simulink model "MMC_SwitchingModel_20250511"  (R2024b)
settings: Solver=VariableStepAuto  StartTime=0.0  StopTime=0.35  RelTol=1e-3
values from neighbouring files (symbols this model uses):
  Ceq = 3e-3    (= 0.003)    [param_allsim_20250429.m]
  f0 = 50    [param_allsim_20250429.m]
  Fc = 1e3    (= 1000)    [param_allsim_20250429.m]
  L_ac = 100e-6    (= 0.0001)    [param_allsim_20250429.m]
  L_arm = 1e-3    (= 0.001)    [param_allsim_20250429.m]
  m_Delta_0 = m_Delta_0_n    (= 0)    [param_allsim_20250429.m]
  m_Delta_d = M_Delta*sin(Phi_Delta)    [param_allsim_20250429.m]
  m_Delta_q = -M_Delta*cos(Phi_Delta)    [param_allsim_20250429.m]
  m_Sigma_0 = m_Sigma_0_n    (= 1)    [param_allsim_20250429.m]
  m_Sigma_d = M_Sigma*sin(Phi_Sigma)    [param_allsim_20250429.m]
  m_Sigma_q = -M_Sigma*cos(Phi_Sigma)    [param_allsim_20250429.m]
  N = 6    [param_allsim_20250429.m]
  R_ac = 1    [param_allsim_20250429.m]
  R_arm = 1e-2    (= 0.01)    [param_allsim_20250429.m]
  VDC = 800    [param_allsim_20250429.m]
undefined symbols (not defined in the file or in its folder): C_SM
libraries: spsVoltageMeasurementLib x11, spsCurrentMeasurementLib x8, spsSeriesRLCBranchLib x6, spsHalfBridgeMMCLib x6, spsPWMGeneratorMultilevelLib x6, spsabctodq0Lib x6, spsDCVoltageSourceLib x2, spsdq0toabcLib x2, spsGroundLib x1, spsThreePhaseSeriesRLCBranchLib x1, spsMeanLib x1, spspowerguiLib x1
(part 2 of 2)

== matlab function MMC_SwitchingModel_20250511/ /Sinus Modulation + Sorting Algorithm/Subsystem3/MATLAB Function1 ==
  data: ordre input; y output; sens input; N_on input
function y = fcn(ordre,sens,N_on)

N_m = length(ordre);
Gp = zeros(1,2*N_m);
Ap0=ordre;

%% Sens positif (sens = 1)
if sens==1         % ON les condensateurs les moins chargés
    
    %K1 = 1 ; K2 = 0
    kp = 1:N_on;
    Gp(2*Ap0(kp))=0;
    Gp(2*Ap0(kp)-1)=1;
    
    %K1 = 0 ; K2 = 1
    kp = N_on+1:N_m;
    Gp(2*Ap0(kp))=1;
    Gp(2*Ap0(kp)-1)=0;

else            % ON les condensateurs les plus chargés
    
    %K1 = 1 ; K2 = 0
    kp = N_m:-1:N_m+1-N_on;
    Gp(2*Ap0(kp))=0;
    Gp(2*Ap0(kp)-1)=1;
    
    %K1 = 0 ; K2 = 1
    kp = N_m-N_on:-1:1;
    Gp(2*Ap0(kp))=1;
    Gp(2*Ap0(kp)-1)=0;
end
y=Gp;

== matlab function MMC_SwitchingModel_20250511/ /Sinus Modulation + Sorting Algorithm/Subsystem3/MATLAB Function2 ==
  data: ordre input; y output; sens input; N_on input
function y = fcn(ordre,sens,N_on)

N_m = length(ordre);
Gp = zeros(1,2*N_m);
Ap0=ordre;

%% Sens positif (sens = 1)
if sens==1         % ON les condensateurs les moins chargés
    
    %K1 = 1 ; K2 = 0
    kp = 1:N_on;
    Gp(2*Ap0(kp))=0;
    Gp(2*Ap0(kp)-1)=1;
    
    %K1 = 0 ; K2 = 1
    kp = N_on+1:N_m;
    Gp(2*Ap0(kp))=1;
    Gp(2*Ap0(kp)-1)=0;

else            % ON les condensateurs les plus chargés
    
    %K1 = 1 ; K2 = 0
    kp = N_m:-1:N_m+1-N_on;
    Gp(2*Ap0(kp))=0;
    Gp(2*Ap0(kp)-1)=1;
    
    %K1 = 0 ; K2 = 1
    kp = N_m-N_on:-1:1;
    Gp(2*Ap0(kp))=1;
    Gp(2*Ap0(kp)-1)=0;
end
y=Gp;

== matlab function MMC_SwitchingModel_20250511/ /Sinus Modulation + Sorting Algorithm/Number_of_Module_to_SWITCH/MATLAB Function2 ==
  data: Nu output; P input
function Nu = fcn(P)

s=0;

for k = 1:2:length(P)
    s=s+P(k);
end

Nu=s;

== matlab function MMC_SwitchingModel_20250511/ /Sinus Modulation + Sorting Algorithm/Number_of_Module_to_SWITCH/MATLAB Function6 ==
  data: Nu output; P input
function Nu = fcn(P)

s=0;

for k = 1:2:length(P)
    s=s+P(k);
end

Nu=s;

== matlab function MMC_SwitchingModel_20250511/ /Sinus Modulation + Sorting Algorithm/Number_of_Module_to_SWITCH/MATLAB Function3 ==
  data: Nu output; P input
function Nu = fcn(P)

s=0;

for k = 1:2:length(P)
    s=s+P(k);
end

Nu=s;

== matlab function MMC_SwitchingModel_20250511/ /Sinus Modulation + Sorting Algorithm/Subsystem1/Tri phase/Tri2 ==
  data: ordre output; Vcp input; i input; sens output
function [ordre,sens] = fcn(Vcp, i)

[~, ordre] = sort(Vcp);

if i > 0 
    sens = 1;
else 
    sens = 0;
end
